simulink model "LLCRE_RESONATOR"  (R2025a)
settings: Solver=VariableStepAuto  StartTime=0.0  StopTime=0.04  RelTol=1e-3
libraries: spsSeriesRLCBranchLib x5, spsDiodeLib x4, spsCurrentMeasurementLib x3, spsMosfetLib x2, spsDCVoltageSourceLib x1, spsLinearTransformerLib x1, spsVoltageMeasurementLib x1, sps_lib x1
settings Model: Creator=VICTUS  LastModifiedBy=VICTUS

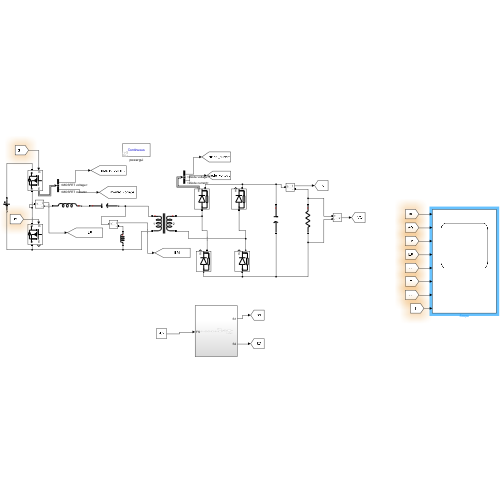
[thumbnail: Simulink's stored preview of the top-level diagram]
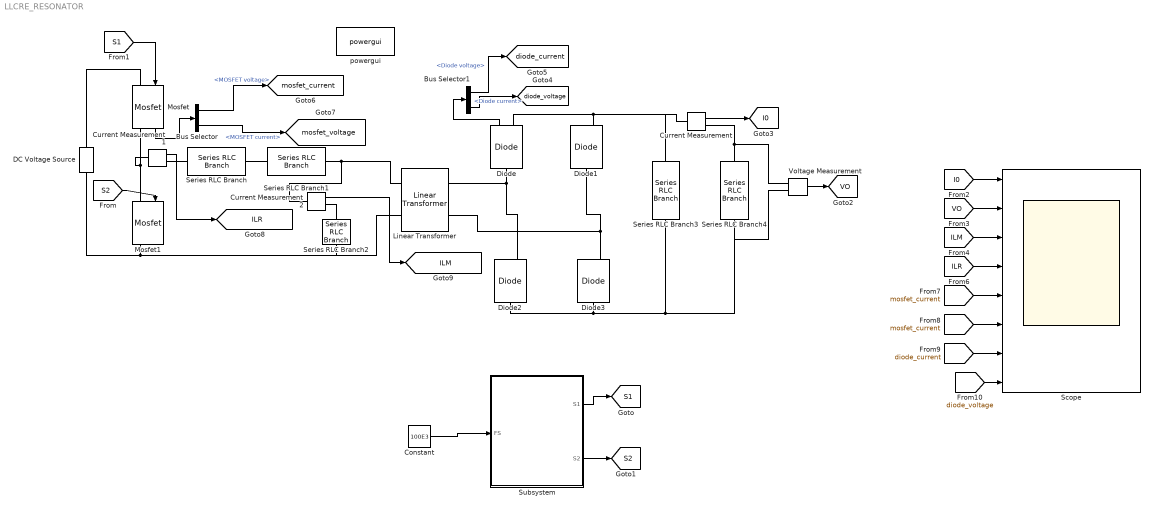
== system LLCRE_RESONATOR ==
  Bus Selector : BusSelector  OutputSignals=MOSFET voltage,MOSFET current
  Bus Selector1 : BusSelector  OutputSignals=Diode voltage,Diode current
  Constant : Constant  Value=100E3
  Current Measurement : spsCurrentMeasurementLib/Current Measurement  PhasorSimulation=off  OutputType=Complex  PSBequivalent=0
  Current Measurement1 : spsCurrentMeasurementLib/Current Measurement  PhasorSimulation=off  OutputType=Complex  PSBequivalent=0
  Current Measurement2 : spsCurrentMeasurementLib/Current Measurement  PhasorSimulation=off  OutputType=Complex  PSBequivalent=0
  DC Voltage Source : spsDCVoltageSourceLib/DC Voltage Source  Amplitude=390  Measurements=None
  Diode{,1..3} (4 alike) : spsDiodeLib/Diode  Ron=0.001  Lon=0  Vf=0.8  IC=0  UseSnubber=0  Rs=500  Cs=250e-9  Measurements=on
  Linear Transformer : spsLinearTransformerLib/Linear Transformer  UNITS=SI  NominalPower=[ 700 100E3 ]  winding1=[3.39 0 0]  winding2=[1 0 0]  ThreeWindings=off  winding3=[3.15e+05 0.7938 0.084225]  RmLm=[100 0]  Measurements=None  DataType=on
  Mosfet : spsMosfetLib/Mosfet  Ron=0.1  Lon=0  Rd=0.01  Vfd=0  IC=0  Rs=1e5  Cs=inf  Measurements=on
  Mosfet1 : spsMosfetLib/Mosfet  Ron=0.1  Lon=0  Rd=0.01  Vfd=0  IC=0  Rs=1e5  Cs=inf  Measurements=on
  Scope : Scope  NumInputPorts=8
      settings: ActiveDisplayYMinimum=11.676892257343685  ActiveDisplayYMaximum=11.717625893898012
  Series RLC Branch : spsSeriesRLCBranchLib/Series RLC Branch  LConnTagsString=__new0  RConnTagsString=__new0  BranchType=L  Resistance=1  Inductance=22e-6  SetiL0=off  InitialCurrent=0  Capacitance=1e-6  Setx0=off  InitialVoltage=0  Measurements=None
  Series RLC Branch1 : spsSeriesRLCBranchLib/Series RLC Branch  LConnTagsString=__new0  RConnTagsString=__new0  BranchType=C  Resistance=1  Inductance=1e-3  SetiL0=off  InitialCurrent=0  Capacitance=112E-9  Setx0=off  InitialVoltage=0  Measurements=None
  Series RLC Branch2 : spsSeriesRLCBranchLib/Series RLC Branch  LConnTagsString=__new0  RConnTagsString=__new0  BranchType=L  Resistance=1  Inductance=3.5*22E-6  SetiL0=off  InitialCurrent=0  Capacitance=1e-6  Setx0=off  InitialVoltage=0  Measurements=None
  Series RLC Branch3 : spsSeriesRLCBranchLib/Series RLC Branch  LConnTagsString=__new0  RConnTagsString=__new0  BranchType=C  Resistance=1  Inductance=1e-3  SetiL0=off  InitialCurrent=0  Capacitance=100e-6  Setx0=off  InitialVoltage=0  Measurements=None
  Series RLC Branch4 : spsSeriesRLCBranchLib/Series RLC Branch  LConnTagsString=__new0  RConnTagsString=__new0  BranchType=R  Resistance=4.833  Inductance=1e-3  SetiL0=off  InitialCurrent=0  Capacitance=1e-6  Setx0=off  InitialVoltage=0  Measurements=None
  Subsystem : Subsystem
  Voltage Measurement : spsVoltageMeasurementLib/Voltage Measurement  PhasorSimulation=off  OutputType=Complex  PSBequivalent=0
  powergui : sps_lib/powergui  Priority=1  SimulationMode=Continuous  SampleTime=50e-6  frequency=60  Iterations=50  frequencyindice=0  Pbase=100e6  ErrMax=1e-4  UnitsV=kV  UnitsW=MW  buscounter=0  FunctionMessages=off  echomessages=off  EnableUseOfTLC=off  CurrentSourceSwitches=off  DisableSnubberDevices=off  DisableRonSwitches=off  DisableVfSwitches=off  DisplayEquations=off  AutomaticDiscreteSolvers=off  SolverType=Tustin/Backward Euler (TBE)  Interpol=off  ExternalGateDelay=off  methode=off  Ts=100  x0status=blocks  SPID=on  SwTol=0  HookPort=off  NonlinearTolerance=1e-4  nMaxIteration=100  ContinueOnMaxIteration=off  RestoreLinks=warning  ResistiveCurrentMeasurement=off  Frange=[0:2:500]  Ylog=off  Xlog=on  ShowGrid=off  save=off  variable=ZData  structure=0  ZoomFFT=off  StartTime=0.0  cycles=1  DisplayStyle=1  fundamental=60  FreqAxis=off  MaxFrequency=1000  frequencyindicesteady=1  RmsSteady=1  display=off
  tag scope: I0=global, ILM=global, ILR=global, S1=global, S2=global, VO=global, diode_current=global, diode_voltage=global, mosfet_current=global, mosfet_voltage=global
  wires:
  Subsystem/2(S2) -> [S2]
  Subsystem/1(S1) -> [S1]
  [S1] -> Mosfet/1
  [S2] -> Mosfet1/1
  Constant/1 -> Subsystem/1(FS)
  Mosfet/1 -> Bus Selector/1
  Diode/1 -> Bus Selector1/1
  Voltage Measurement/1 -> [VO]
  Current Measurement/1 -> [I0]
  Bus Selector1/1 -> [diode_current]  "<Diode voltage>"
  Bus Selector1/2 -> [diode_voltage]  "<Diode current>"
  Bus Selector/1 -> [mosfet_current]  "<MOSFET voltage>"
  Bus Selector/2 -> [mosfet_voltage]  "<MOSFET current>"
  Current Measurement1/1 -> [ILR]
  Current Measurement2/1 -> [ILM]
  [I0] -> Scope/1
  [diode_voltage] -> Scope/8
  [diode_current] -> Scope/7
  [mosfet_current] -> Scope/6
  [mosfet_current] -> Scope/5
  [ILR] -> Scope/4
  [ILM] -> Scope/3
  [VO] -> Scope/2
  connections:
  DC Voltage Source/RConn1 -- Mosfet/LConn1
  DC Voltage Source/LConn1 -- Linear Transformer/LConn2 -- Series RLC Branch2/RConn1 -- Mosfet1/RConn1
  Mosfet/RConn1 -- Current Measurement1/LConn1 -- Mosfet1/LConn1
  Series RLC Branch/LConn1 -- Series RLC Branch1/LConn1
  Linear Transformer/LConn1 -- Current Measurement2/LConn1 -- Series RLC Branch1/RConn1
  Diode/LConn1 -- Linear Transformer/RConn1 -- Diode2/RConn1
  Diode1/LConn1 -- Diode3/RConn1 -- Linear Transformer/RConn2
  Diode2/LConn1 -- Voltage Measurement/LConn2 -- Series RLC Branch4/RConn1 -- Series RLC Branch3/RConn1 -- Diode3/LConn1
  Diode/RConn1 -- Series RLC Branch3/LConn1 -- Current Measurement/LConn1 -- Diode1/RConn1
  Current Measurement/RConn1 -- Voltage Measurement/LConn1 -- Series RLC Branch4/LConn1
  Current Measurement1/RConn1 -- Series RLC Branch/RConn1
  Current Measurement2/RConn1 -- Series RLC Branch2/LConn1

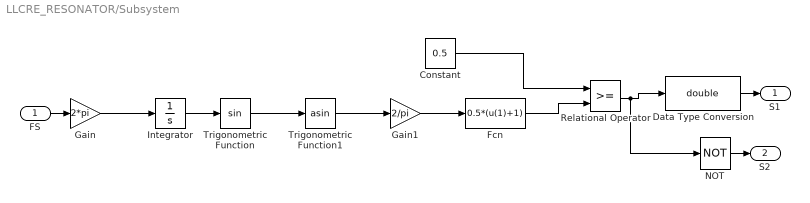
== system LLCRE_RESONATOR/Subsystem ==
  FS : Inport
  Constant : Constant  Value=0.5
  Data Type Conversion : DataTypeConversion  OutDataTypeStr=double  SaturateOnIntegerOverflow=off  RndMeth=Floor
  Fcn : Fcn  Expr=0.5*(u(1)+1)
  Gain : Gain  Gain=2*pi
  Gain1 : Gain  Gain=2/pi
  Integrator : Integrator
  NOT : Logic  Operator=NOT  IconShape=distinctive  AllPortsSameDT=off  OutDataTypeStr=boolean
  Relational Operator : RelationalOperator  OutDataTypeStr=boolean  RndMeth=Simplest  InputSameDT=off
  Trigonometric Function : Trigonometry
  Trigonometric Function1 : Trigonometry  Operator=asin
  S1 : Outport
  S2 : Outport  Port=2
  wires:
  Relational Operator/1 -> NOT/1, Data Type Conversion/1
  Gain/1 -> Integrator/1
  Trigonometric Function/1 -> Trigonometric Function1/1
  Integrator/1 -> Trigonometric Function/1
  Constant/1 -> Relational Operator/1
  FS/1 -> Gain/1
  Gain1/1 -> Fcn/1
  Trigonometric Function1/1 -> Gain1/1
  Fcn/1 -> Relational Operator/2
  NOT/1 -> S2/1
  Data Type Conversion/1 -> S1/1
